simulink model "Model_1"  (R2020b)
settings: Solver=VariableStepAuto  StartTime=0.0  StopTime=10.0  RelTol=1e-3
settings Model: Creator=Akarsh  LastModifiedBy=Akarsh

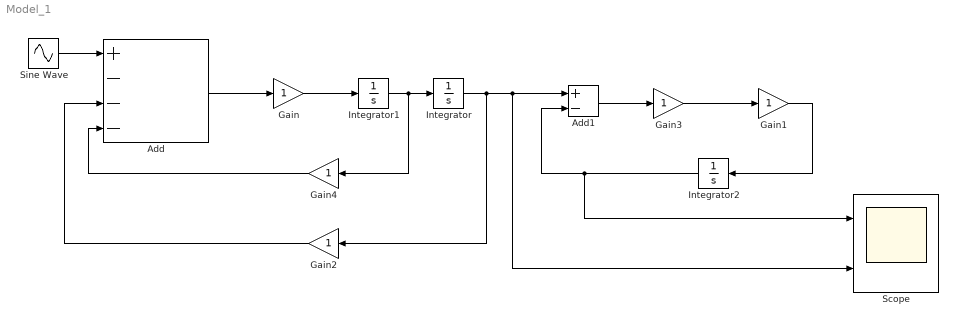
== system Model_1 ==
  Add : Sum  Inputs=+---
  Add1 : Sum  Inputs=+-
  Gain{,1..4} (5 alike) : Gain
  Integrator : Integrator
  Integrator1 : Integrator
  Integrator2 : Integrator
  Scope : Scope  NumInputPorts=2
  Sine Wave : Sin  Amplitude=2  Frequency=2*pi*10  SampleTime=0
  wires:
  Add/1 -> Gain/1
  Gain/1 -> Integrator1/1
  Integrator1/1 -> Gain4/1, Integrator/1
  Integrator/1 -> Gain2/1, Add1/1, Scope/2
  Add1/1 -> Gain3/1
  Gain3/1 -> Gain1/1
  Gain1/1 -> Integrator2/1
  Integrator2/1 -> Scope/1, Add1/2
  Gain4/1 -> Add/4
  Gain2/1 -> Add/3
  Sine Wave/1 -> Add/1
